simulink model "new_nncACCsystem_5_50"  (R2021a)
(part 7 of 14)

  "IW{3,2}(50,:)'" : Constant  Value=[-0.8763858200696807987384318039403297007083892822265625;0.67093832511001583185361596406437456607818603515625;-0.9987327446773850425643104244954884052276611328125;-0.9890923925705512598227642229176126420497894287109375;-0.5300963879799576172757724634720943868160247802734375;0.64516357970568716240222784108482301235198974609375;-0.1191062615841766980651073026820085942745208740234375;-0.4867148110374761582619385080761276185512542724609375;0.1476685048293884250369956134818494319915771484375;0.5033750785207484756966778149944730103015899658203125;0.5892964885570368682721209552255459129810333251953125;0.71207088122677486552447589929215610027313232421875;-0.9345406930662594202630089057493023574352264404296875;-0.9903968018453459531968974260962568223476409912109375;-0.9615471952037728531337279491708613932132720947265625;-0.768718471680795545353248598985373973846435546875;0.4129483945999137262106160051189363002777099609375;0.073574932639954848667684927931986749172210693359375;0.573323458463765422976621266570873558521270751953125;0.2000633364743773512373081757687032222747802734375;0.666770477430901120641237866948358714580535888671875;-0.9929483708686797083231567739858292043209075927734375;0.5783083574000131843462213510065339505672454833984375;0.4608107423098093402558106390642933547496795654296875;-0.39644873351967557795205721049569547176361083984375;-0.1374561743052620244043282582424581050872802734375;-0.2345626744917435058113142076763324439525604248046875;0.365624966622390079606930157751776278018951416015625;-0.1903073743161585174021865896065719425678253173828125;-0.4404281365660889235869035474024713039398193359375;0.99607599241557931435409045661799609661102294921875;-0.263188498243397628328921200591139495372772216796875;-0.523948723358209189626677471096627414226531982421875;-0.0596503003863511072069059082423336803913116455078125;-0.4202994690909809261114560285932384431362152099609375;-0.053522075613378294889344033435918390750885009765625;-0.121430487295230538080659243860282003879547119140625;0.987065045210763880589865948422811925411224365234375;-0.2155185252879470159115271599148400127887725830078125;-0.765455904322333235967334985616616904735565185546875;0.174432757803651750094786621048115193843841552734375;0.917817988316443233998143114149570465087890625;-0.1057514852778831393464997745468281209468841552734375;0.384569015222072874138348197448067367076873779296875;-0.1462729471166064332265932534937746822834014892578125;0.6711722304847784759118667352595366537570953369140625;-0.764962447175938198284939062432385981082916259765625;-0.678595784674528967883588848053477704524993896484375;-0.6309473764901631920309910128707997500896453857421875;0.517580124421557652425462947576306760311126708984375]
      mask Display: e = 0.06;c1 = [120 150 230]/255;c2 = ([120 150 230]+0)/383;c3 = ([120 150 230]+128)/383;patch([0 1 1 0],[0 0 1 1],c1);patch([0 1 1 1-e 1-e 0+e],[0 0 1 1-e 0+e 0+e],c2);patch([0 0 1 1-e 0+e 0+e],[0 1 1 1-e 1-e 0+e],c3);plot([0 1 1 0 0],[0 0 1 1 0]);disp('weights');
  "IW{3,2}(6,:)'" : Constant  Value=[0.038896418707861979413564768037758767604827880859375;-0.192739095759538958674284003791399300098419189453125;-0.3360975012976676890019689381006173789501190185546875;-0.94399681847888405883395535056479275226593017578125;0.09098003019948475156297718058340251445770263671875;0.24656728451580267602594176423735916614532470703125;0.1835026239551982296660526117193512618541717529296875;-0.756332123033521153132596737123094499111175537109375;-0.62732900530858781706911031506024301052093505859375;0.6081831843412108806745663969195447862148284912109375;-0.76271731698001499211159170954488217830657958984375;0.687063127422427921686676199897192418575286865234375;0.6931538067404992009556963239447213709354400634765625;-0.1804475727397558681985856310348026454448699951171875;0.8990823887485819287945787436910904943943023681640625;0.7496452270481930302281625699833966791629791259765625;-0.9813076615087954479577092570252716541290283203125;-0.6398581948435613231396246192161925137042999267578125;0.2925375613150602571721492495271377265453338623046875;-0.91872200623645117190108067006804049015045166015625;-0.35241149673224736460497297230176627635955810546875;-0.293849202975625889422417458263225853443145751953125;0.59550576372267638447510762489400804042816162109375;0.0666843955445226566070004992070607841014862060546875;-0.819239143477187070629952359013259410858154296875;0.7845975487414664772956029992201365530490875244140625;0.2282937289518092160989226613310165703296661376953125;0.1303297746132667800367244126391597092151641845703125;0.16666721398682060595319853746332228183746337890625;-0.9082114829382275100755350649706088006496429443359375;-0.59269456376610829551054848707281053066253662109375;-0.7204487517530215878736044032848440110683441162109375;-0.8261368553590575647405103154596872627735137939453125;-0.836188584965455117270494156400673091411590576171875;-0.0242673842237508541330726075102575123310089111328125;-0.77196023885949660581218267907388508319854736328125;-0.6294970974537188457276215558522380888462066650390625;0.790273047821996588169213282526470720767974853515625;0.7198532716333687631049542687833309173583984375;0.84210577633297578614701706101186573505401611328125;-0.61706913371985461225222024950198829174041748046875;-0.248316466901941534928255350678227841854095458984375;-0.8738385616938424416133557315333746373653411865234375;0.45043889190627250940224257647059857845306396484375;-0.03392195612545645388991033541969954967498779296875;0.691746972825150852060005490784533321857452392578125;-0.2737924268969014196528632965055294334888458251953125;0.68032385839173770136767416261136531829833984375;-0.0923224859755436000341433100402355194091796875;-0.3821802243071845683886067490675486624240875244140625]
      mask Display: e = 0.06;c1 = [120 150 230]/255;c2 = ([120 150 230]+0)/383;c3 = ([120 150 230]+128)/383;patch([0 1 1 0],[0 0 1 1],c1);patch([0 1 1 1-e 1-e 0+e],[0 0 1 1-e 0+e 0+e],c2);patch([0 0 1 1-e 0+e 0+e],[0 1 1 1-e 1-e 0+e],c3);plot([0 1 1 0 0],[0 0 1 1 0]);disp('weights');
  "IW{3,2}(7,:)'" : Constant  Value=[0.49763926141077430287396055064164102077484130859375;0.7913633910176967045657647759071551263332366943359375;-0.5955488524411525208535067577031441032886505126953125;0.9791019890770498168564017760218121111392974853515625;-0.8630652455885952090142154702334664762020111083984375;-0.9989926993884716832639014683081768453121185302734375;0.3829299493117985786483359333942644298076629638671875;-0.8342308664033797338532849607872776687145233154296875;0.2371063199266851828639346422278322279453277587890625;-0.9459061594033519870805548634962178766727447509765625;-0.3197558520751868638143378120730631053447723388671875;0.9532528539363716024723771624849177896976470947265625;-0.065014990299315567057192311040125787258148193359375;0.494610415769225486570803695940412580966949462890625;0.46357899273821434604769819998182356357574462890625;0.1370968412391253554716286089387722313404083251953125;-0.771457708953059206891111898585222661495208740234375;0.819690668194601013141209477907977998256683349609375;-0.0589856815586602412082584123709239065647125244140625;-0.9895120316529053550169692243798635900020599365234375;-0.79793126626112798049916818854399025440216064453125;-0.2325633222599770011385089674149639904499053955078125;0.763715293654832816372390880133025348186492919921875;-0.444206914507881744924588929279707372188568115234375;0.1520454979750198720722664802451618015766143798828125;-0.4403282738911389326830203572171740233898162841796875;0.79187444299524667457035320694558322429656982421875;0.7762543567458111137824516845284961163997650146484375;-0.640193200226240488603934863931499421596527099609375;0.9871921623854564842304171179421246051788330078125;-0.2474804126072058796381725187529809772968292236328125;-0.4068982437995902756711075198836624622344970703125;0.62656077214660488294839524314738810062408447265625;-0.35661595470259310758365245419554412364959716796875;-0.25760874857413984528875516843982040882110595703125;0.4852532333600911851334558377857320010662078857421875;0.480066550577761486096051157801412045955657958984375;-0.619810019967114822492249004426412284374237060546875;0.9191787064313530208892188966274261474609375;0.3148574932857888253323608296341262757778167724609375;-0.3234869376393458839658023862284608185291290283203125;-0.8798048743409727645570228560245595872402191162109375;0.678385418836799036768070436664856970310211181640625;-0.0542054144889367872650609569973312318325042724609375;-0.8785351567095782687744076611124910414218902587890625;0.230461875699769169756336850696243345737457275390625;-0.3453654293979304679140795997227542102336883544921875;-0.8338254779905245328563978546299040317535400390625;-0.5780212289447614892878846148960292339324951171875;-0.0905879886823719449040481777046807110309600830078125]
      mask Display: e = 0.06;c1 = [120 150 230]/255;c2 = ([120 150 230]+0)/383;c3 = ([120 150 230]+128)/383;patch([0 1 1 0],[0 0 1 1],c1);patch([0 1 1 1-e 1-e 0+e],[0 0 1 1-e 0+e 0+e],c2);patch([0 0 1 1-e 0+e 0+e],[0 1 1 1-e 1-e 0+e],c3);plot([0 1 1 0 0],[0 0 1 1 0]);disp('weights');
  "IW{3,2}(8,:)'" : Constant  Value=[0.0368657439658885976996316458098590373992919921875;-0.668825033774560484545190774952061474323272705078125;0.65950663523807129262621629095519892871379852294921875;0.0277983921398142243275319884787677437998354434967041015625;0.65202923835810133734725013709976337850093841552734375;-0.8465301458220222396988674518070183694362640380859375;-0.047289019434995797908083403626733343116939067840576171875;0.57032067310396616921508439190802164375782012939453125;0.1999233823314072455712420151030528359115123748779296875;0.2944299529319547303884974098764359951019287109375;0.6456017147730077621048394576064310967922210693359375;0.392326186416664557388145340155460871756076812744140625;-0.53805195965079111175555226509459316730499267578125;-0.330645501146598352892880257059005089104175567626953125;-0.10703643573611475170448414928614511154592037200927734375;-0.5859489732580858145638558198697865009307861328125;-0.1476761029346904674497409359901212155818939208984375;0.155181496420392139867772129946388304233551025390625;0.4034962799173162917298895990825258195400238037109375;0.1369538052051810506082318852349999360740184783935546875;0.25078700274859022645301820375607348978519439697265625;-0.10868922947632746189849939355553942732512950897216796875;-0.41953532532452531000899398350156843662261962890625;0.286205546802082377855214190276456065475940704345703125;0.401880547275501431858657497286912985146045684814453125;-0.61091242817396518294259522008360363543033599853515625;0.85186926770914495055109227905631996691226959228515625;0.7505071971403918240639541181735694408416748046875;0.0885560499848825621871384328187559731304645538330078125;-0.5679852061803842833143107782234437763690948486328125;0.34988681060717119475356184921110980212688446044921875;-0.774213465568557968055074525182135403156280517578125;-0.1643153129847017002163056531571783125400543212890625;-0.0175095982950264072997015318833291530609130859375;-0.614620476025873330172544228844344615936279296875;-0.704196152098231831217844955972395837306976318359375;0.98726599680975102302227242034859955310821533203125;0.782715807922326423096137659740634262561798095703125;0.1984212562034772531216475499604712240397930145263671875;0.7990729865761296846216055200784467160701751708984375;0.35622379368221912532277428908855654299259185791015625;-0.50083065927976366804585950376349501311779022216796875;0.9608127089353419858497318273293785750865936279296875;-0.0662244257173474348832087343907915055751800537109375;-0.90674695402960736601016833446919918060302734375;0.89367169053722594895816655480302870273590087890625;-0.922440256369492228571971281780861318111419677734375;0.07594824659290584645265909102818113751709461212158203125;0.03363557592561594589142259792424738407135009765625;0.499538208331333333234169913339428603649139404296875]
      mask Display: e = 0.06;c1 = [120 150 230]/255;c2 = ([120 150 230]+0)/383;c3 = ([120 150 230]+128)/383;patch([0 1 1 0],[0 0 1 1],c1);patch([0 1 1 1-e 1-e 0+e],[0 0 1 1-e 0+e 0+e],c2);patch([0 0 1 1-e 0+e 0+e],[0 1 1 1-e 1-e 0+e],c3);plot([0 1 1 0 0],[0 0 1 1 0]);disp('weights');
  "IW{3,2}(9,:)'" : Constant  Value=[0.7372101016783216831385061595938168466091156005859375;-0.453647217014030434967253313516266644001007080078125;-0.8377025033846425827732673496939241886138916015625;-0.39737631170325027341050372342579066753387451171875;0.7465522351333635509007535802084021270275115966796875;-0.5957705389561152031774327042512595653533935546875;0.3791919260855693973866209489642642438411712646484375;-0.624400801228033319745236440212465822696685791015625;-0.013289289186799724262755262316204607486724853515625;-0.5041652032579164721681763694505207240581512451171875;-0.1231979304956010157212631384027190506458282470703125;-0.1131925383884031521830593192134983837604522705078125;-0.9409258076441080476115530473180115222930908203125;-0.788300403034450258843435221933759748935699462890625;-0.6569493945828244196860623560496605932712554931640625;-0.3612481456114748912256118273944593966007232666015625;0.8108543186368886157566748806857503950595855712890625;-0.02091102480974971200566869811154901981353759765625;-0.0907669981552221560860971294459886848926544189453125;-0.492024952160486694907604032778181135654449462890625;0.8986542128253576233731791944592259824275970458984375;0.8751732151200288800652060672291554510593414306640625;0.7046545809127191528631328765186481177806854248046875;-0.5897840766816944135797484705108217895030975341796875;0.667176876824743914085047435946762561798095703125;-0.6994112892134349834805107093416154384613037109375;-0.50929835525626998560255742631852626800537109375;-0.0319717626878439631354922312311828136444091796875;-0.4065998616798236486857831550878472626209259033203125;0.39654334288107850881033300538547337055206298828125;-0.2614973163449423321225140171009115874767303466796875;0.155269258066373705418072859174571931362152099609375;0.556895883758861121037853081361390650272369384765625;0.551803600351379319732814110466279089450836181640625;0.301269034832944537782850602525286376476287841796875;0.547545079995087835555978017509914934635162353515625;0.496158656492929228676302955136634409427642822265625;-0.638733832948029434106729240738786756992340087890625;0.165381398799007595101784318103455007076263427734375;-0.7170376752291056643429101313813589513301849365234375;0.617796149586677056930739126983098685741424560546875;-0.2299380883228010485908043847302906215190887451171875;0.6066565013062403810550904381670989096164703369140625;-0.5098856297925185021568950105574913322925567626953125;-0.0277077691471754317120712585165165364742279052734375;-0.3157516326225735525667914771474897861480712890625;-0.3205998371598555163330956929712556302547454833984375;-0.7585294451305528706797076665679924190044403076171875;0.0561658873750736642449510327423922717571258544921875;-0.98931444254884848277242781477980315685272216796875]
      mask Display: e = 0.06;c1 = [120 150 230]/255;c2 = ([120 150 230]+0)/383;c3 = ([120 150 230]+128)/383;patch([0 1 1 0],[0 0 1 1],c1);patch([0 1 1 1-e 1-e 0+e],[0 0 1 1-e 0+e 0+e],c2);patch([0 0 1 1-e 0+e 0+e],[0 1 1 1-e 1-e 0+e],c3);plot([0 1 1 0 0],[0 0 1 1 0]);disp('weights');
  Mux : Mux  Inputs=50
      mask Display: e = 0.06;c1 = [120 150 230]/255;c2 = ([120 150 230]+0)/383;c3 = ([120 150 230]+128)/383;patch([0 1 1 0],[0 0 1 1],c1);patch([0 1 1 1-e 1-e 0+e],[0 0 1 1-e 0+e 0+e],c2);patch([0 0 1 1-e 0+e 0+e],[0 1 1 1-e 1-e 0+e],c3);plot([0 1 1 0 0],[0 0 1 1 0]);disp('Mux');
  dotprod{1..50} (50 alike) : neural/Weight Functions/dotprod
  "lz{3,2}" : Outport
      mask Display: e = 0.06;c1 = [120 230 180]/255;c2 = ([120 230 180]+0)/(256+128);c3 = ([120 230 180]+128)/(256+128);patch([0 1 1 0],[0 0 1 1],c1);patch([0 1 1 1-e 1-e 0+e],[0 0 1 1-e 0+e 0+e],c2);patch([0 0 1 1-e 0+e 0+e],[0 1 1 1-e 1-e 0+e],c3);plot([0 1 1 0 0],[0 0 1 1 0]);
  wires:
  "IW{3,2}(1,:)'"/1 -> dotprod1/1
  "ad{3,2}"/1 -> dotprod1/2, dotprod2/2, dotprod3/2, dotprod4/2, dotprod5/2, dotprod6/2, dotprod7/2, dotprod8/2, dotprod9/2, dotprod10/2, dotprod11/2, dotprod12/2, dotprod13/2, dotprod14/2, dotprod15/2, dotprod16/2, dotprod17/2, dotprod18/2, dotprod19/2, dotprod20/2, dotprod21/2, dotprod22/2, dotprod23/2, dotprod24/2, dotprod25/2, dotprod26/2, dotprod27/2, dotprod28/2, dotprod29/2, dotprod30/2, dotprod31/2, dotprod32/2, dotprod33/2, dotprod34/2, dotprod35/2, dotprod36/2, dotprod37/2, dotprod38/2, dotprod39/2, dotprod40/2, dotprod41/2, dotprod42/2, dotprod43/2, dotprod44/2, dotprod45/2, dotprod46/2, dotprod47/2, dotprod48/2, dotprod49/2, dotprod50/2
  dotprod1/1 -> Mux/1
  "IW{3,2}(2,:)'"/1 -> dotprod2/1
  dotprod2/1 -> Mux/2
  "IW{3,2}(3,:)'"/1 -> dotprod3/1
  dotprod3/1 -> Mux/3
  "IW{3,2}(4,:)'"/1 -> dotprod4/1
  dotprod4/1 -> Mux/4
  "IW{3,2}(5,:)'"/1 -> dotprod5/1
  dotprod5/1 -> Mux/5
  "IW{3,2}(6,:)'"/1 -> dotprod6/1
  dotprod6/1 -> Mux/6
  "IW{3,2}(7,:)'"/1 -> dotprod7/1
  dotprod7/1 -> Mux/7
  "IW{3,2}(8,:)'"/1 -> dotprod8/1
  dotprod8/1 -> Mux/8
  "IW{3,2}(9,:)'"/1 -> dotprod9/1
  dotprod9/1 -> Mux/9
  "IW{3,2}(10,:)'"/1 -> dotprod10/1
  dotprod10/1 -> Mux/10
  "IW{3,2}(11,:)'"/1 -> dotprod11/1
  dotprod11/1 -> Mux/11
  "IW{3,2}(12,:)'"/1 -> dotprod12/1
  dotprod12/1 -> Mux/12
  "IW{3,2}(13,:)'"/1 -> dotprod13/1
  dotprod13/1 -> Mux/13
  "IW{3,2}(14,:)'"/1 -> dotprod14/1
  dotprod14/1 -> Mux/14
  "IW{3,2}(15,:)'"/1 -> dotprod15/1
  dotprod15/1 -> Mux/15
  "IW{3,2}(16,:)'"/1 -> dotprod16/1
  dotprod16/1 -> Mux/16
  "IW{3,2}(17,:)'"/1 -> dotprod17/1
  dotprod17/1 -> Mux/17
  "IW{3,2}(18,:)'"/1 -> dotprod18/1
  dotprod18/1 -> Mux/18
  "IW{3,2}(19,:)'"/1 -> dotprod19/1
  dotprod19/1 -> Mux/19
  "IW{3,2}(20,:)'"/1 -> dotprod20/1
  dotprod20/1 -> Mux/20
  "IW{3,2}(21,:)'"/1 -> dotprod21/1
  dotprod21/1 -> Mux/21
  "IW{3,2}(22,:)'"/1 -> dotprod22/1
  dotprod22/1 -> Mux/22
  "IW{3,2}(23,:)'"/1 -> dotprod23/1
  dotprod23/1 -> Mux/23
  "IW{3,2}(24,:)'"/1 -> dotprod24/1
  dotprod24/1 -> Mux/24
  "IW{3,2}(25,:)'"/1 -> dotprod25/1
  dotprod25/1 -> Mux/25
  "IW{3,2}(26,:)'"/1 -> dotprod26/1
  dotprod26/1 -> Mux/26
  "IW{3,2}(27,:)'"/1 -> dotprod27/1
  dotprod27/1 -> Mux/27
  "IW{3,2}(28,:)'"/1 -> dotprod28/1
  dotprod28/1 -> Mux/28
  "IW{3,2}(29,:)'"/1 -> dotprod29/1
  dotprod29/1 -> Mux/29
  "IW{3,2}(30,:)'"/1 -> dotprod30/1
  dotprod30/1 -> Mux/30
  "IW{3,2}(31,:)'"/1 -> dotprod31/1
  dotprod31/1 -> Mux/31
  "IW{3,2}(32,:)'"/1 -> dotprod32/1
  dotprod32/1 -> Mux/32
  "IW{3,2}(33,:)'"/1 -> dotprod33/1
  dotprod33/1 -> Mux/33
  "IW{3,2}(34,:)'"/1 -> dotprod34/1
  dotprod34/1 -> Mux/34
  "IW{3,2}(35,:)'"/1 -> dotprod35/1
  dotprod35/1 -> Mux/35
  "IW{3,2}(36,:)'"/1 -> dotprod36/1
  dotprod36/1 -> Mux/36
  "IW{3,2}(37,:)'"/1 -> dotprod37/1
  dotprod37/1 -> Mux/37
  "IW{3,2}(38,:)'"/1 -> dotprod38/1
  dotprod38/1 -> Mux/38
  "IW{3,2}(39,:)'"/1 -> dotprod39/1
  dotprod39/1 -> Mux/39
  "IW{3,2}(40,:)'"/1 -> dotprod40/1
  dotprod40/1 -> Mux/40
  "IW{3,2}(41,:)'"/1 -> dotprod41/1
  dotprod41/1 -> Mux/41
  "IW{3,2}(42,:)'"/1 -> dotprod42/1
  dotprod42/1 -> Mux/42
  "IW{3,2}(43,:)'"/1 -> dotprod43/1
  dotprod43/1 -> Mux/43
  "IW{3,2}(44,:)'"/1 -> dotprod44/1
  dotprod44/1 -> Mux/44
  "IW{3,2}(45,:)'"/1 -> dotprod45/1
  dotprod45/1 -> Mux/45
  "IW{3,2}(46,:)'"/1 -> dotprod46/1
  dotprod46/1 -> Mux/46
  "IW{3,2}(47,:)'"/1 -> dotprod47/1
  dotprod47/1 -> Mux/47
  "IW{3,2}(48,:)'"/1 -> dotprod48/1
  dotprod48/1 -> Mux/48
  "IW{3,2}(49,:)'"/1 -> dotprod49/1
  dotprod49/1 -> Mux/49
  "IW{3,2}(50,:)'"/1 -> dotprod50/1
  dotprod50/1 -> Mux/50
  Mux/1 -> "lz{3,2}"/1
